simulink model "UnitTest_relay_R25SyncCheck"  (Simulink 8.1)
settings: Solver=ode4  StartTime=0.0  StopTime=.7  FixedStep=Ts  MaxStep=1e-3  RelTol=1e-3
model workspace (MAT data in the model file):
  op_snapshot1 : opcond.OperatingPoint (value not decoded)
PostLoadFcn:
  | Ts=100e-6;
InitFcn:
  | Ts=100e-6;
libraries: powerlib x3, breaker_lib x1, relay_ANSI_F25_lib x1, powerlib_extras x1
settings Model: ARTEMISmethode_block_infos=$$__separator__$$  Creator=RE25624  LastModifiedBy=re25624  BufferReuse=off
settings SolverCC: ZeroCrossAlgorithm=Adaptive
settings DataIOCC: ExternalInput=getinputstruct(op_snapshot1)  InitialState=getstatestruct(op_snapshot1)  LimitDataPoints=off  MaxDataPoints=90060  SignalLoggingSaveFormat=Dataset  SaveOutput=off  SignalLogging=off  DSMLogging=off  SaveTime=off  OutputSaveName=result
settings OptimizationCC: BlockReduction=off  OptimizeBlockIOStorage=off  BufferReuse=off  ExpressionFolding=off  LocalBlockOutputs=off
settings DebuggingCC: MaxConsecutiveZCsMsg=warning  IgnoredZcDiagnostic=none  SolverPrmCheckMsg=none  MultiTaskRateTransMsg=warning  FcnCallInpInsideContextMsg=EnableAllAsWarning  FrameProcessingCompatibilityMsg=error  ModelReferenceExtraNoncontSigs=warning  StrictBusMsg=None
settings ModelReferenceCC: UpdateModelReferenceTargets=IfOutOfDate
settings SFSimCC: SFSimEcho=off
settings GRTTargetCC: CodeReplacementLibrary=C89/C90 (ANSI)

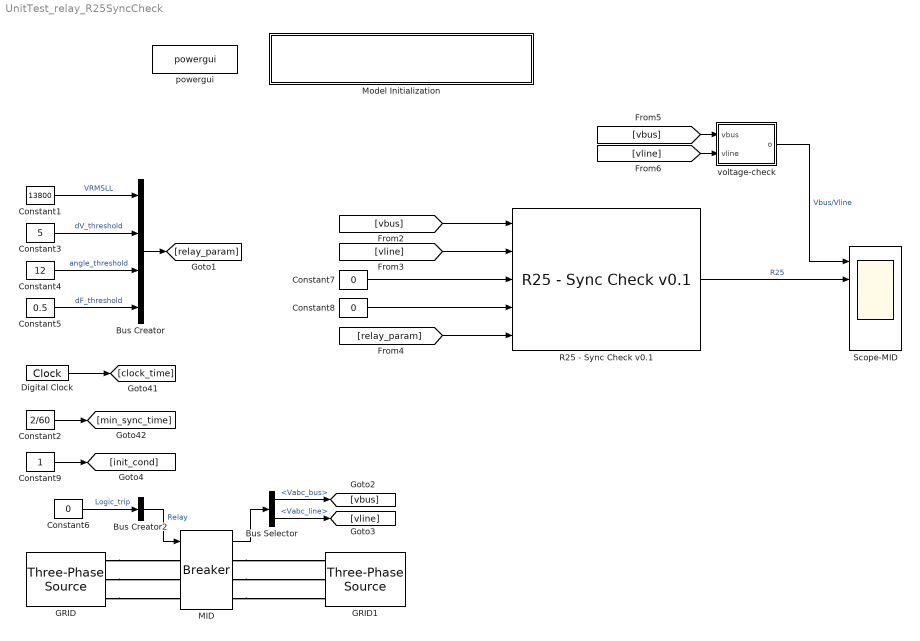
== system UnitTest_relay_R25SyncCheck ==
  Bus Creator : BusCreator
  Bus Creator2 : BusCreator  Inputs=1
  Bus Selector : BusSelector  OutputSignals=Vabc_bus,Vabc_line
  Constant1 : Constant  Value=13800
  Constant2 : Constant  Value=2/60
  Constant3 : Constant  Value=5
  Constant4 : Constant  Value=12
  Constant5 : Constant  Value=0.5
  Constant6 : Constant  Value=0
  Constant7 : Constant  Value=0
  Constant8 : Constant  Value=0
  Constant9 : Constant
  Digital Clock : DigitalClock  SampleTime=Ts
  GRID : powerlib/Electrical Sources/Three-Phase Source  Voltage=13800 * 1.0  PhaseAngle=0  Frequency=60  InternalConnection=Yg  SpecifyImpedance=on  Resistance=0.8929  Inductance=16.58e-3  ShortCircuitLevel=375e6  BaseVoltage=13800  XRratio=7.9  BusType=swing  Pref=0  Qref=0  Qmin=-inf  Qmax=inf
  GRID1 : powerlib/Electrical Sources/Three-Phase Source  Voltage=13800 * 1.1  PhaseAngle=0  Frequency=60  InternalConnection=Yg  SpecifyImpedance=on  Resistance=0.8929  Inductance=16.58e-3  ShortCircuitLevel=375e6  BaseVoltage=13800  XRratio=7.9  BusType=swing  Pref=0  Qref=0  Qmin=-inf  Qmax=inf
  MID : breaker_lib/Breaker  Ts=Ts  mech_delays=[5 5] ./ 60
  Model Initialization : Subsystem  AncestorBlock=artemis/Tools /Misc/Model Initialization  mask(Model Functions){InitFcnX=Ts=100e-6;, prel=off, posl=on, inif=on, strf=off}
      mask prompts: InitFcnX "Initialisation"; prel "Preload Function"; posl "PostLoad Function"; inif "InitFcn"; strf "StartFcn"
      mask init:
      | currentBlock = gcb;
      | root = bdroot(currentBlock);
      | 
      | 
      | if ~strcmp(get_param(root,'BlockDiagramType'),'library')
      |     if prel==1
      |         set_param(root, 'PreLoadFcn', InitFcnX);
      |     else
      |         set_param(root, 'PreLoadFcn', '');
      |     end
      |     if inif==1
      |         set_param(root, 'InitFcn', InitFcnX);
      |     else
      |         set_param(root, 'InitFcn', '');
      |     end
      |     if strf==1
      |         set_param(root, 'StartFcn', InitFcnX);
      |     else
      |         set_param(root, 'StartFcn', '');
      |     end
      |     if posl==1
      |         set_param(root, 'PostLoadFcn', InitFcnX);
      |     else
      |         set_param(root, 'PostLoadFcn', '');
      |     end
      | end
      | 
      | pos = get_param(currentBlock, 'Position');
      | width = pos(3) - pos(1); height = pos(4) - pos(2);
      | txt = [ upper(root) '\n' '- InitFcn. . . . . '  get_param(root, 'InitFcn') ];
      settings: CopyFcn=set_param(gcb,'LinkStatus','inactive')
      mask Display: text(5, height*0.5, txt, 'horizontalAlignment', 'left', 'verticalAlignment', 'middle') ;
  R25 - Sync Check v0.1 : relay_ANSI_F25_lib/R25 - Sync Check v0.1  Ts=Ts
  Scope-MID : Scope  NumInputPorts=5
      settings: TimeRange=0.7000000000000001  YMin=0.8~-1~-1~-1~-1  YMax=1.15~1.5~1~1~1  SaveName=ScopeData4
  powergui : powerlib/powergui  Priority=2  SimulationMode=Discrete  SolverType=Tustin  SampleTime=Ts  frequency=60  SPID=off  DisableSnubberDevices=off  DisableRonSwitches=off  DisableVfSwitches=off  SwTol=0  Interpol=off  DisplayEquations=off  frequencyindice=0  Pbase=100e6  ErrMax=1e-4  Iterations=50  UnitsV=kV  UnitsW=MW  FunctionMessages=off  echomessages=off  HookPort=off  EnableUseOfTLC=off  x0status=blocks  RestoreLinks=warning  ResistiveCurrentMeasurement=off  Frange=logspace(0,3,50)  Ylog=off  Xlog=off  ShowGrid=off  save=off  variable=ZData  structure=0  ZoomFFT=on  StartTime=0.0  cycles=2  DisplayStyle=off  fundamental=60  FreqAxis=off  MaxFrequency=1000  frequencyindicesteady=1  RmsSteady=1  display=off  Ts=0  methode=off
  voltage-check : Subsystem
  wires:
  Digital Clock/1 -> [clock_time]
  Constant2/1 -> [min_sync_time]
  Constant1/1 -> Bus Creator/1  "VRMSLL"
  Constant4/1 -> Bus Creator/3  "angle_threshold"
  Constant3/1 -> Bus Creator/2  "dV_threshold"
  Constant5/1 -> Bus Creator/4  "dF_threshold"
  Bus Creator/1 -> [relay_param]
  MID/1 -> Bus Selector/1
  Bus Creator2/1 -> MID/1  "Relay"
  Constant6/1 -> Bus Creator2/1  "Logic_trip"
  Bus Selector/1 -> [vbus]  "<Vabc_bus>"
  Bus Selector/2 -> [vline]  "<Vabc_line>"
  [vbus] -> R25 - Sync Check v0.1/1
  [vline] -> R25 - Sync Check v0.1/2
  Constant7/1 -> R25 - Sync Check v0.1/3
  Constant8/1 -> R25 - Sync Check v0.1/4
  [relay_param] -> R25 - Sync Check v0.1/5
  R25 - Sync Check v0.1/1 -> Scope-MID/2  "R25"
  [vbus] -> voltage-check/1(vbus)
  [vline] -> voltage-check/2(vline)
  voltage-check/1(o) -> Scope-MID/1  "Vbus/Vline"
  Constant9/1 -> [init_cond]
  connections:
  GRID/RConn2 -- MID/LConn2
  GRID/RConn1 -- MID/LConn1
  GRID/RConn3 -- MID/LConn3
  MID/RConn2 -- GRID1/RConn2
  MID/RConn3 -- GRID1/RConn3
  MID/RConn1 -- GRID1/RConn1

== system UnitTest_relay_R25SyncCheck/Model Initialization ==

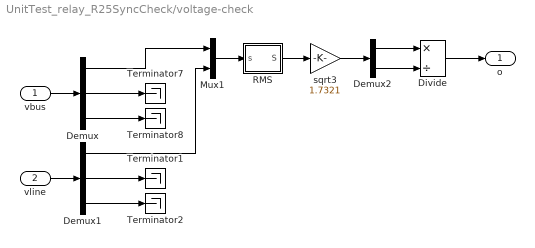
== system UnitTest_relay_R25SyncCheck/voltage-check ==
  vbus : Inport
  vline : Inport  Port=2
  Demux : Demux  Outputs=3
  Demux1 : Demux  Outputs=3
  Demux2 : Demux  Outputs=2
  Divide : Product  Inputs=*/
  Mux1 : Mux  Inputs=2
  RMS : Subsystem
  Terminator{1..2,7..8} (4 alike) : Terminator
  sqrt3 : Gain  Gain=1.7321
  o : Outport
  wires:
  Demux2/1 -> Divide/1
  Divide/1 -> o/1
  Demux2/2 -> Divide/2
  Demux1/2 -> Terminator1/1
  Demux1/1 -> Mux1/2
  Demux1/3 -> Terminator2/1
  Mux1/1 -> RMS/1(s)
  sqrt3/1 -> Demux2/1
  RMS/1(S) -> sqrt3/1
  Demux/3 -> Terminator8/1
  Demux/1 -> Mux1/1
  Demux/2 -> Terminator7/1
  vline/1 -> Demux1/1
  vbus/1 -> Demux/1

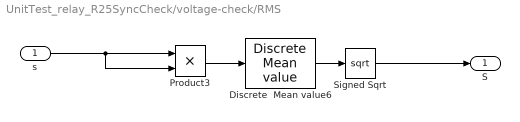
== system UnitTest_relay_R25SyncCheck/voltage-check/RMS ==
  s : Inport
  Discrete  Mean value6 : powerlib_extras/Discrete Measurements/Discrete  Mean value  Freq=60  Vinit=0  Ts=Ts
  Product3 : Product  RndMeth=Zero
  Signed Sqrt : Sqrt  SaturateOnIntegerOverflow=on
  S : Outport
  wires:
  Signed Sqrt/1 -> S/1
  Discrete  Mean value6/1 -> Signed Sqrt/1
  Product3/1 -> Discrete  Mean value6/1
  s/1 -> Product3/2, Product3/1
